simulink model "DroneSubsystem"  (R2018b)
settings: Solver=VariableStepAuto  StartTime=0.0  StopTime=10  RelTol=1e-3
values from neighbouring files (symbols this model uses):
  Ax = [0 1  0   0 ... (first row only)    [DroneSubsystemModelling.m]
  Ay = [0 1  0   0 ... (first row only)    [DroneSubsystemModelling.m]
  Bx = [0;0;0;b1]    [DroneSubsystemModelling.m]
  By = [0;0;0;b2]    [DroneSubsystemModelling.m]
  Cpx = [1 0 0 0]    [DroneSubsystemModelling.m]
  Cpy = [1 0 0 0]    [DroneSubsystemModelling.m]
  Cvx = [0 1 0 0]    [DroneSubsystemModelling.m]
  Cvy = [0 1 0 0]    [DroneSubsystemModelling.m]
  Dx = zeros(1,1)    [DroneSubsystemModelling.m]
  Dy = zeros(1,1)    [DroneSubsystemModelling.m]
  Ts = 0.001    [DroneSubsystemModelling.m]
  X40 = [x40 vx40 0 0]'    [MotionModelling.m]
  Y40 = [y40 vy40 0 0]'    [MotionModelling.m]
undefined symbols (not defined in the file or in its folder): x0, y0
libraries: simulink x6
settings Model: Creator=CowUser  LastModifiedBy=CowUser

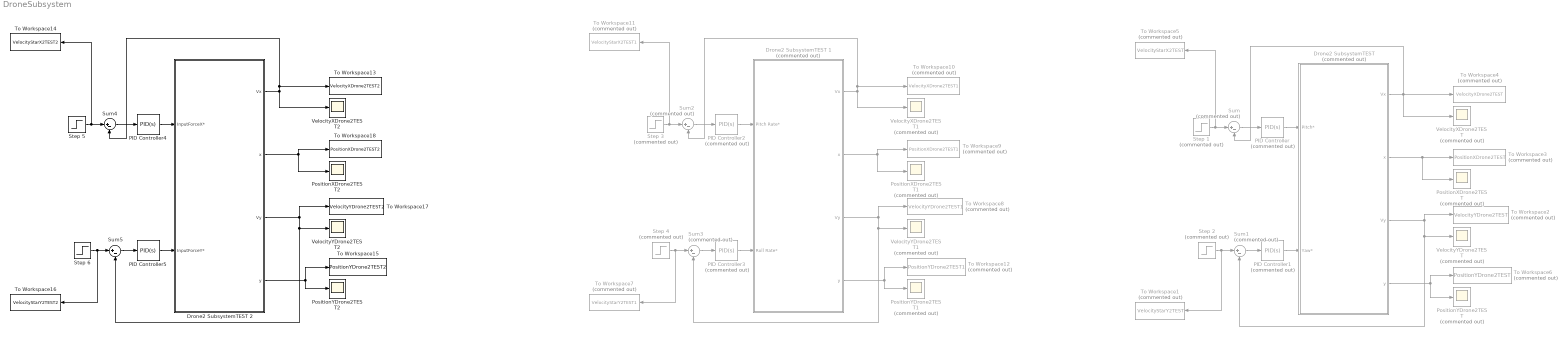
== system DroneSubsystem ==
  "Drone2 SubsystemTEST " : Subsystem  Commented=on
  Drone2 SubsystemTEST 1 : Subsystem  Commented=on
  Drone2 SubsystemTEST 2 : Subsystem
  PID Controller{,1..3} (4 alike) : simulink/Continuous/PID Controller  Commented=on  Controller=PID  Form=Parallel  TimeDomain=Continuous-time  SampleTime=-1  IntegratorMethod=Forward Euler  FilterMethod=Forward Euler  ControllerParametersSource=internal  P=800  I=40  D=1  UseFilter=on  N=100  TunerSelectOption=Transfer Function Based (PID Tuner App)  InitialConditionSource=internal  InitialConditionForIntegrator=0  InitialConditionForFilter=0  DifferentiatorICPrevScaledInput=0  ExternalReset=none  TrackingMode=off  Kt=1  LimitOutput=off  UpperSaturationLimit=inf  LowerSaturationLimit=-inf  LinearizeAsGain=on  AntiWindupMode=none  Kb=1  POutMin=[]  POutMax=[]  IOutMin=[]  IOutMax=[]  DOutMin=[]  DOutMax=[]  NOutMin=[]  NOutMax=[]  SumOutMin=[]  SumOutMax=[]  SaturationOutMin=[]  SaturationOutMax=[]  PParamMin=[]  PParamMax=[]  IParamMin=[]  IParamMax=[]  DParamMin=[]  DParamMax=[]  NParamMin=[]  NParamMax=[]  KbParamMin=[]  KbParamMax=[]  KtParamMin=[]  KtParamMax=[]  KbOutMin=[]  KbOutMax=[]  KtOutMin=[]  KtOutMax=[]  IntegratorOutMin=[]  IntegratorOutMax=[]  FilterOutMin=[]  FilterOutMax=[]  SumI1OutMin=[]  SumI1OutMax=[]  SumI2OutMin=[]  SumI2OutMax=[]  SumI3OutMin=[]  SumI3OutMax=[]  SumI4OutMin=[]  SumI4OutMax=[]  SumDOutMin=[]  SumDOutMax=[]  DifferentiatorOutMin=[]  DifferentiatorOutMax=[]  FilterDiffOutCoefMin=[]  FilterDiffOutCoefMax=[]  ReciprocalOutMin=[]  ReciprocalOutMax=[]  SumDenOutMin=[]  SumDenOutMax=[]  SumNumOutMin=[]  SumNumOutMax=[]  DivideOutMin=[]  DivideOutMax=[]  IntegratorContinuousStateAttributes=''  IntegratorStateMustResolveToSignalObject=off  IntegratorRTWStateStorageClass=Auto  FilterContinuousStateAttributes=''  FilterStateMustResolveToSignalObject=off  FilterRTWStateStorageClass=Auto  ParallelPVariant=InternalParameters  IdealPVariant=Disabled  IVariant=InternalParameters  DVariant=InternalParameters  IntegratorVariant=Continuous  SatVariant=Disabled  AWVariant=Passthrough  PCopyVariant=Disabled  TRVariant=Disabled  FdbkBlocksVariant=Forward  IdealPFdbkVariant=Disabled  SatFdbkVariant=Disabled  DerivativeFilterVariant=ContFilter  NVariant=InternalParameters  NCopyVariant=Disabled  FilterICVariant=InternalICsFilter  IntegratorICVariant=InternalICs  ExternalResetVariant=Disabled  TRSumVariant=Passthrough  SumFdbkVariant=Disabled  SumVariant=Sum_PID
  PID Controller4 : simulink/Continuous/PID Controller  Controller=PID  Form=Parallel  TimeDomain=Continuous-time  SampleTime=-1  IntegratorMethod=Forward Euler  FilterMethod=Forward Euler  ControllerParametersSource=internal  P=0.193233207738566  I=0.0113997087231983  D=0.323760304852997  UseFilter=on  N=866.923674741149  TunerSelectOption=Transfer Function Based (PID Tuner App)  InitialConditionSource=internal  InitialConditionForIntegrator=0  InitialConditionForFilter=0  DifferentiatorICPrevScaledInput=0  ExternalReset=none  TrackingMode=off  Kt=1  LimitOutput=off  UpperSaturationLimit=inf  LowerSaturationLimit=-inf  LinearizeAsGain=on  AntiWindupMode=none  Kb=1  POutMin=[]  POutMax=[]  IOutMin=[]  IOutMax=[]  DOutMin=[]  DOutMax=[]  NOutMin=[]  NOutMax=[]  SumOutMin=[]  SumOutMax=[]  SaturationOutMin=[]  SaturationOutMax=[]  PParamMin=[]  PParamMax=[]  IParamMin=[]  IParamMax=[]  DParamMin=[]  DParamMax=[]  NParamMin=[]  NParamMax=[]  KbParamMin=[]  KbParamMax=[]  KtParamMin=[]  KtParamMax=[]  KbOutMin=[]  KbOutMax=[]  KtOutMin=[]  KtOutMax=[]  IntegratorOutMin=[]  IntegratorOutMax=[]  FilterOutMin=[]  FilterOutMax=[]  SumI1OutMin=[]  SumI1OutMax=[]  SumI2OutMin=[]  SumI2OutMax=[]  SumI3OutMin=[]  SumI3OutMax=[]  SumI4OutMin=[]  SumI4OutMax=[]  SumDOutMin=[]  SumDOutMax=[]  DifferentiatorOutMin=[]  DifferentiatorOutMax=[]  FilterDiffOutCoefMin=[]  FilterDiffOutCoefMax=[]  ReciprocalOutMin=[]  ReciprocalOutMax=[]  SumDenOutMin=[]  SumDenOutMax=[]  SumNumOutMin=[]  SumNumOutMax=[]  DivideOutMin=[]  DivideOutMax=[]  IntegratorContinuousStateAttributes=''  IntegratorStateMustResolveToSignalObject=off  IntegratorRTWStateStorageClass=Auto  FilterContinuousStateAttributes=''  FilterStateMustResolveToSignalObject=off  FilterRTWStateStorageClass=Auto  ParallelPVariant=InternalParameters  IdealPVariant=Disabled  IVariant=InternalParameters  DVariant=InternalParameters  IntegratorVariant=Continuous  SatVariant=Disabled  AWVariant=Passthrough  PCopyVariant=Disabled  TRVariant=Disabled  FdbkBlocksVariant=Forward  IdealPFdbkVariant=Disabled  SatFdbkVariant=Disabled  DerivativeFilterVariant=ContFilter  NVariant=InternalParameters  NCopyVariant=Disabled  FilterICVariant=InternalICsFilter  IntegratorICVariant=InternalICs  ExternalResetVariant=Disabled  TRSumVariant=Passthrough  SumFdbkVariant=Disabled  SumVariant=Sum_PID
  PID Controller5 : simulink/Continuous/PID Controller  Controller=PID  Form=Parallel  TimeDomain=Continuous-time  SampleTime=-1  IntegratorMethod=Forward Euler  FilterMethod=Forward Euler  ControllerParametersSource=internal  P=1.97139727738968e-05  I=1.5233344900537e-08  D=0.00566857635684116  UseFilter=on  N=15.1370363747334  TunerSelectOption=Transfer Function Based (PID Tuner App)  InitialConditionSource=internal  InitialConditionForIntegrator=0  InitialConditionForFilter=0  DifferentiatorICPrevScaledInput=0  ExternalReset=none  TrackingMode=off  Kt=1  LimitOutput=off  UpperSaturationLimit=inf  LowerSaturationLimit=-inf  LinearizeAsGain=on  AntiWindupMode=none  Kb=1  POutMin=[]  POutMax=[]  IOutMin=[]  IOutMax=[]  DOutMin=[]  DOutMax=[]  NOutMin=[]  NOutMax=[]  SumOutMin=[]  SumOutMax=[]  SaturationOutMin=[]  SaturationOutMax=[]  PParamMin=[]  PParamMax=[]  IParamMin=[]  IParamMax=[]  DParamMin=[]  DParamMax=[]  NParamMin=[]  NParamMax=[]  KbParamMin=[]  KbParamMax=[]  KtParamMin=[]  KtParamMax=[]  KbOutMin=[]  KbOutMax=[]  KtOutMin=[]  KtOutMax=[]  IntegratorOutMin=[]  IntegratorOutMax=[]  FilterOutMin=[]  FilterOutMax=[]  SumI1OutMin=[]  SumI1OutMax=[]  SumI2OutMin=[]  SumI2OutMax=[]  SumI3OutMin=[]  SumI3OutMax=[]  SumI4OutMin=[]  SumI4OutMax=[]  SumDOutMin=[]  SumDOutMax=[]  DifferentiatorOutMin=[]  DifferentiatorOutMax=[]  FilterDiffOutCoefMin=[]  FilterDiffOutCoefMax=[]  ReciprocalOutMin=[]  ReciprocalOutMax=[]  SumDenOutMin=[]  SumDenOutMax=[]  SumNumOutMin=[]  SumNumOutMax=[]  DivideOutMin=[]  DivideOutMax=[]  IntegratorContinuousStateAttributes=''  IntegratorStateMustResolveToSignalObject=off  IntegratorRTWStateStorageClass=Auto  FilterContinuousStateAttributes=''  FilterStateMustResolveToSignalObject=off  FilterRTWStateStorageClass=Auto  ParallelPVariant=InternalParameters  IdealPVariant=Disabled  IVariant=InternalParameters  DVariant=InternalParameters  IntegratorVariant=Continuous  SatVariant=Disabled  AWVariant=Passthrough  PCopyVariant=Disabled  TRVariant=Disabled  FdbkBlocksVariant=Forward  IdealPFdbkVariant=Disabled  SatFdbkVariant=Disabled  DerivativeFilterVariant=ContFilter  NVariant=InternalParameters  NCopyVariant=Disabled  FilterICVariant=InternalICsFilter  IntegratorICVariant=InternalICs  ExternalResetVariant=Disabled  TRSumVariant=Passthrough  SumFdbkVariant=Disabled  SumVariant=Sum_PID
  PositionXDrone2TEST : Scope  Commented=on
  PositionXDrone2TEST1 : Scope  Commented=on
  PositionXDrone2TEST2 : Scope
  PositionYDrone2TEST : Scope  Commented=on
  PositionYDrone2TEST1 : Scope  Commented=on
  PositionYDrone2TEST2 : Scope
  Step {1..4} (4 alike) : Step  Commented=on  Time=0  After=-0.1061  SampleTime=0
  Step 5 : Step  Time=0  After=0.1061  SampleTime=0
  Step 6 : Step  Time=0  After=0.1061  SampleTime=0
  Sum{,1..3} (4 alike) : Sum  Commented=on  Inputs=|+-
  Sum4 : Sum  Inputs=|+-
  Sum5 : Sum  Inputs=|+-
  To Workspace1 : ToWorkspace  Commented=on  VariableName=VelocityStarY2TEST  SampleTime=-1
  To Workspace10 : ToWorkspace  Commented=on  VariableName=VelocityXDrone2TEST1  SampleTime=-1
  To Workspace11 : ToWorkspace  Commented=on  VariableName=VelocityStarX2TEST1  SampleTime=-1
  To Workspace12 : ToWorkspace  Commented=on  VariableName=PositionYDrone2TEST1  SampleTime=-1
  To Workspace13 : ToWorkspace  VariableName=VelocityXDrone2TEST2  SampleTime=-1
  To Workspace14 : ToWorkspace  VariableName=VelocityStarX2TEST2  SampleTime=-1
  To Workspace15 : ToWorkspace  VariableName=PositionYDrone2TEST2  SampleTime=-1
  To Workspace16 : ToWorkspace  VariableName=VelocityStarY2TEST2  SampleTime=-1
  To Workspace17 : ToWorkspace  VariableName=VelocityYDrone2TEST2  SampleTime=-1
  To Workspace18 : ToWorkspace  VariableName=PositionXDrone2TEST2  SampleTime=-1
  To Workspace2 : ToWorkspace  Commented=on  VariableName=VelocityYDrone2TEST  SampleTime=-1
  To Workspace3 : ToWorkspace  Commented=on  VariableName=PositionXDrone2TEST  SampleTime=-1
  To Workspace4 : ToWorkspace  Commented=on  VariableName=VelocityXDrone2TEST  SampleTime=-1
  To Workspace5 : ToWorkspace  Commented=on  VariableName=VelocityStarX2TEST  SampleTime=-1
  To Workspace6 : ToWorkspace  Commented=on  VariableName=PositionYDrone2TEST  SampleTime=-1
  To Workspace7 : ToWorkspace  Commented=on  VariableName=VelocityStarY2TEST1  SampleTime=-1
  To Workspace8 : ToWorkspace  Commented=on  VariableName=VelocityYDrone2TEST1  SampleTime=-1
  To Workspace9 : ToWorkspace  Commented=on  VariableName=PositionXDrone2TEST1  SampleTime=-1
  VelocityXDrone2TEST : Scope  Commented=on
  VelocityXDrone2TEST1 : Scope  Commented=on
  VelocityXDrone2TEST2 : Scope
  VelocityYDrone2TEST : Scope  Commented=on
  VelocityYDrone2TEST1 : Scope  Commented=on
  VelocityYDrone2TEST2 : Scope
  wires:
  Step 2/1 -> To Workspace1/1, Sum1/1
  "Drone2 SubsystemTEST "/2(x) -> To Workspace3/1, PositionXDrone2TEST/1
  Sum1/1 -> PID Controller1/1
  PID Controller/1 -> "Drone2 SubsystemTEST "/1(Pitch*)
  Sum/1 -> PID Controller/1
  "Drone2 SubsystemTEST "/4(y) -> To Workspace6/1, PositionYDrone2TEST/1
  PID Controller1/1 -> "Drone2 SubsystemTEST "/2("Yaw* ")
  Step 1/1 -> Sum/1, To Workspace5/1
  "Drone2 SubsystemTEST "/3(Vy) -> To Workspace2/1, Sum1/2, VelocityYDrone2TEST/1
  "Drone2 SubsystemTEST "/1(Vx) -> VelocityXDrone2TEST/1, Sum/2, To Workspace4/1
  Sum3/1 -> PID Controller3/1
  Step 4/1 -> To Workspace7/1, Sum3/1
  Step 3/1 -> Sum2/1, To Workspace11/1
  PID Controller3/1 -> Drone2 SubsystemTEST 1/2("Roll Rate* ")
  Drone2 SubsystemTEST 1/1(Vx) -> Sum2/2, To Workspace10/1, VelocityXDrone2TEST1/1
  Drone2 SubsystemTEST 1/4(y) -> To Workspace12/1, PositionYDrone2TEST1/1
  Drone2 SubsystemTEST 1/2(x) -> To Workspace9/1, PositionXDrone2TEST1/1
  Drone2 SubsystemTEST 1/3(Vy) -> Sum3/2, VelocityYDrone2TEST1/1, To Workspace8/1
  Sum2/1 -> PID Controller2/1
  PID Controller2/1 -> Drone2 SubsystemTEST 1/1(Pitch Rate*)
  Sum4/1 -> PID Controller4/1
  Drone2 SubsystemTEST 2/1(Vx) -> Sum4/2, To Workspace13/1, VelocityXDrone2TEST2/1
  Drone2 SubsystemTEST 2/2(x) -> To Workspace18/1, PositionXDrone2TEST2/1
  PID Controller4/1 -> Drone2 SubsystemTEST 2/1(InputForceX*)
  Step 5/1 -> Sum4/1, To Workspace14/1
  Sum5/1 -> PID Controller5/1
  Drone2 SubsystemTEST 2/3(Vy) -> Sum5/2, VelocityYDrone2TEST2/1, To Workspace17/1
  Drone2 SubsystemTEST 2/4(y) -> To Workspace15/1, PositionYDrone2TEST2/1
  Step 6/1 -> To Workspace16/1, Sum5/1
  PID Controller5/1 -> Drone2 SubsystemTEST 2/2("InputForceY* ")

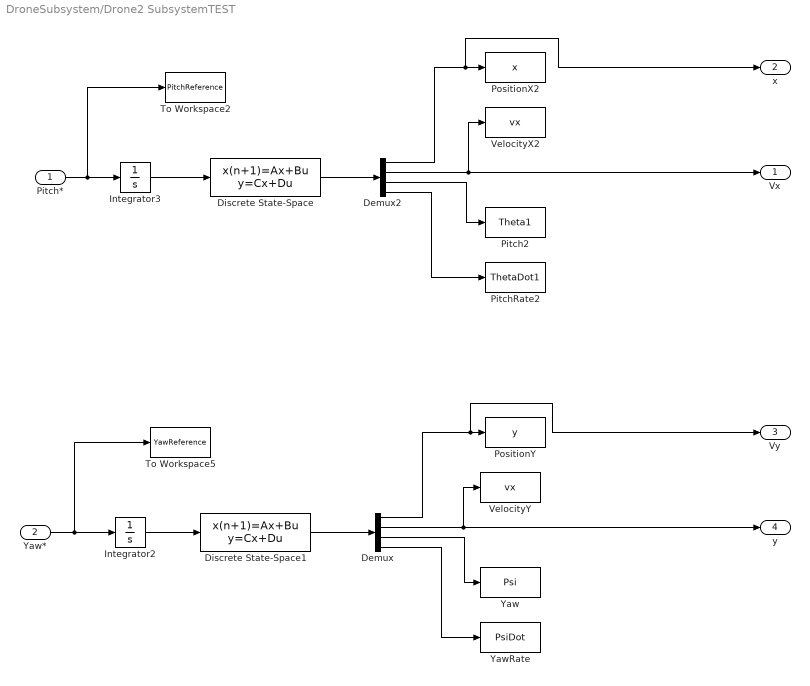
== system DroneSubsystem/Drone2 SubsystemTEST  ==
  Pitch* : Inport
  "Yaw* " : Inport  Port=2
  Demux : Demux
  Demux2 : Demux
  Discrete State-Space : DiscreteStateSpace  A=Ax  B=Bx  C=Cvx  D=Dx  InitialCondition=x0  SampleTime=Ts
  Discrete State-Space1 : DiscreteStateSpace  A=Ay  B=By  C=Cvy  D=Dy  InitialCondition=y0  SampleTime=Ts
  Integrator2 : Integrator
  Integrator3 : Integrator
  Pitch2 : ToWorkspace  VariableName=Theta1  SampleTime=-1
  PitchRate2 : ToWorkspace  VariableName=ThetaDot1  SampleTime=-1
  PositionX2 : ToWorkspace  VariableName=x  SampleTime=-1
  PositionY : ToWorkspace  VariableName=y  SampleTime=-1
  To Workspace2 : ToWorkspace  VariableName=PitchReference  SampleTime=-1
  To Workspace5 : ToWorkspace  VariableName=YawReference  SampleTime=-1
  VelocityX2 : ToWorkspace  VariableName=vx  SampleTime=-1
  VelocityY : ToWorkspace  VariableName=vx  SampleTime=-1
  Yaw : ToWorkspace  VariableName=Psi  SampleTime=-1
  YawRate : ToWorkspace  VariableName=PsiDot  SampleTime=-1
  Vx : Outport
  x : Outport  Port=2
  Vy : Outport  Port=3
  y : Outport  Port=4
  wires:
  Integrator3/1 -> Discrete State-Space/1
  Pitch*/1 -> Integrator3/1, To Workspace2/1
  Demux2/3 -> Pitch2/1
  Discrete State-Space/1 -> Demux2/1
  Demux2/4 -> PitchRate2/1
  Integrator2/1 -> Discrete State-Space1/1
  "Yaw* "/1 -> Integrator2/1, To Workspace5/1
  Demux/3 -> Yaw/1
  Discrete State-Space1/1 -> Demux/1
  Demux/4 -> YawRate/1
  Demux2/2 -> Vx/1, VelocityX2/1
  Demux2/1 -> x/1, PositionX2/1
  Demux/2 -> VelocityY/1, y/1
  Demux/1 -> Vy/1, PositionY/1

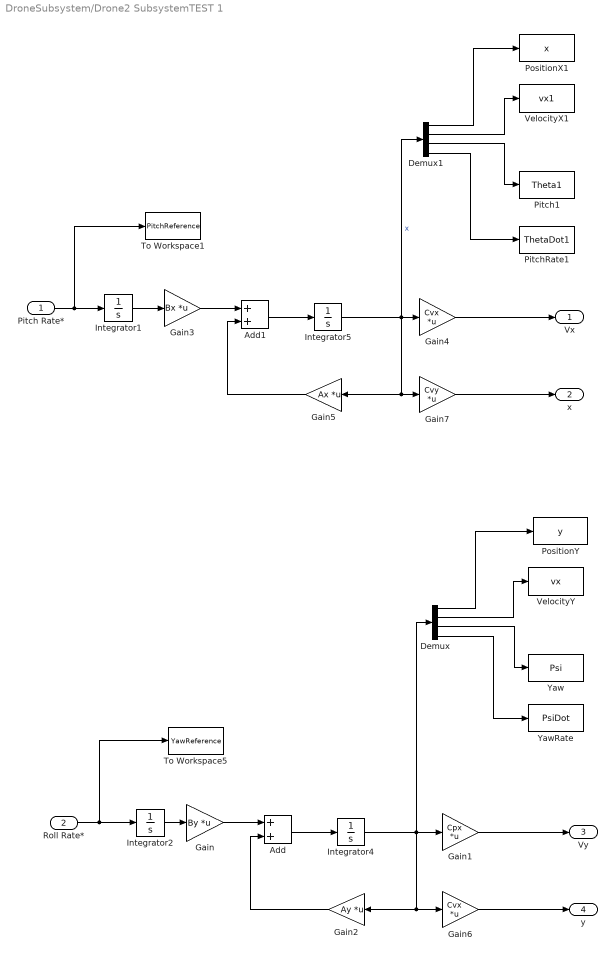
== system DroneSubsystem/Drone2 SubsystemTEST 1 ==
  Pitch Rate* : Inport
  "Roll Rate* " : Inport  Port=2
  Add : Sum
  Add1 : Sum
  Demux : Demux
  Demux1 : Demux
  Gain : Gain  Gain=By  Multiplication=Matrix(K*u)
  Gain1 : Gain  Gain=Cpx  Multiplication=Matrix(K*u)
  Gain2 : Gain  Gain=Ay  Multiplication=Matrix(K*u)
  Gain3 : Gain  Gain=Bx  Multiplication=Matrix(K*u)
  Gain4 : Gain  Gain=Cvx  Multiplication=Matrix(K*u)
  Gain5 : Gain  Gain=Ax  Multiplication=Matrix(K*u)
  Gain6 : Gain  Gain=Cvx  Multiplication=Matrix(K*u)
  Gain7 : Gain  Gain=Cvy  Multiplication=Matrix(K*u)
  Integrator1 : Integrator
  Integrator2 : Integrator
  Integrator4 : Integrator  InitialCondition=y0
  Integrator5 : Integrator  InitialCondition=x0
  Pitch1 : ToWorkspace  VariableName=Theta1  SampleTime=-1
  PitchRate1 : ToWorkspace  VariableName=ThetaDot1  SampleTime=-1
  PositionX1 : ToWorkspace  VariableName=x  SampleTime=-1
  PositionY : ToWorkspace  VariableName=y  SampleTime=-1
  To Workspace1 : ToWorkspace  VariableName=PitchReference  SampleTime=-1
  To Workspace5 : ToWorkspace  VariableName=YawReference  SampleTime=-1
  VelocityX1 : ToWorkspace  VariableName=vx1  SampleTime=-1
  VelocityY : ToWorkspace  VariableName=vx  SampleTime=-1
  Yaw : ToWorkspace  VariableName=Psi  SampleTime=-1
  YawRate : ToWorkspace  VariableName=PsiDot  SampleTime=-1
  Vx : Outport
  x : Outport  Port=2
  Vy : Outport  Port=3
  y : Outport  Port=4
  wires:
  Demux1/4 -> PitchRate1/1
  Demux1/2 -> VelocityX1/1
  Integrator2/1 -> Gain/1
  Gain4/1 -> Vx/1
  Integrator1/1 -> Gain3/1
  Integrator4/1 -> Gain6/1, Gain2/1, Demux/1, Gain1/1
  Integrator5/1 -> Gain4/1, Gain5/1, Gain7/1, Demux1/1  "x"
  Add1/1 -> Integrator5/1
  Gain5/1 -> Add1/2
  Demux1/3 -> Pitch1/1
  Gain3/1 -> Add1/1
  Gain7/1 -> x/1
  Pitch Rate*/1 -> Integrator1/1, To Workspace1/1
  Gain2/1 -> Add/2
  Demux/2 -> VelocityY/1
  Gain1/1 -> Vy/1
  Add/1 -> Integrator4/1
  Demux1/1 -> PositionX1/1
  Gain6/1 -> y/1
  Demux/3 -> Yaw/1
  Demux/1 -> PositionY/1
  "Roll Rate* "/1 -> Integrator2/1, To Workspace5/1
  Gain/1 -> Add/1
  Demux/4 -> YawRate/1

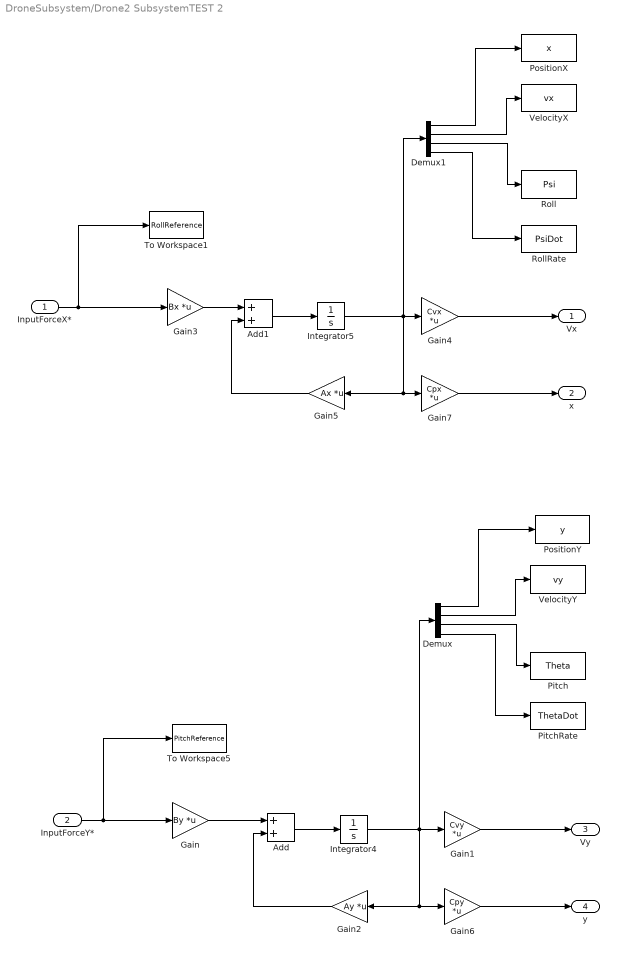
== system DroneSubsystem/Drone2 SubsystemTEST 2 ==
  InputForceX* : Inport
  "InputForceY* " : Inport  Port=2
  Add : Sum
  Add1 : Sum
  Demux : Demux
  Demux1 : Demux
  Gain : Gain  Gain=By  Multiplication=Matrix(K*u)
  Gain1 : Gain  Gain=Cvy  Multiplication=Matrix(K*u)
  Gain2 : Gain  Gain=Ay  Multiplication=Matrix(K*u)
  Gain3 : Gain  Gain=Bx  Multiplication=Matrix(K*u)
  Gain4 : Gain  Gain=Cvx  Multiplication=Matrix(K*u)
  Gain5 : Gain  Gain=Ax  Multiplication=Matrix(K*u)
  Gain6 : Gain  Gain=Cpy  Multiplication=Matrix(K*u)
  Gain7 : Gain  Gain=Cpx  Multiplication=Matrix(K*u)
  Integrator4 : Integrator  InitialCondition=Y40
  Integrator5 : Integrator  InitialCondition=X40
  Pitch : ToWorkspace  VariableName=Theta  SampleTime=-1
  PitchRate : ToWorkspace  VariableName=ThetaDot  SampleTime=-1
  PositionX : ToWorkspace  VariableName=x  SampleTime=-1
  PositionY : ToWorkspace  VariableName=y  SampleTime=-1
  Roll : ToWorkspace  VariableName=Psi  SampleTime=-1
  RollRate : ToWorkspace  VariableName=PsiDot  SampleTime=-1
  To Workspace1 : ToWorkspace  VariableName=RollReference  SampleTime=-1
  To Workspace5 : ToWorkspace  VariableName=PitchReference  SampleTime=-1
  VelocityX : ToWorkspace  VariableName=vx  SampleTime=-1
  VelocityY : ToWorkspace  VariableName=vy  SampleTime=-1
  Vx : Outport
  x : Outport  Port=2
  Vy : Outport  Port=3
  y : Outport  Port=4
  wires:
  Demux1/4 -> RollRate/1
  Demux1/2 -> VelocityX/1
  Gain4/1 -> Vx/1
  Integrator4/1 -> Gain6/1, Gain2/1, Demux/1, Gain1/1
  Integrator5/1 -> Gain4/1, Gain5/1, Gain7/1, Demux1/1
  Add1/1 -> Integrator5/1
  Gain5/1 -> Add1/2
  Demux1/3 -> Roll/1
  Gain3/1 -> Add1/1
  Gain7/1 -> x/1
  Gain2/1 -> Add/2
  Demux/2 -> VelocityY/1
  Gain1/1 -> Vy/1
  Add/1 -> Integrator4/1
  Demux1/1 -> PositionX/1
  Gain6/1 -> y/1
  Demux/3 -> Pitch/1
  Demux/1 -> PositionY/1
  Gain/1 -> Add/1
  Demux/4 -> PitchRate/1
  "InputForceY* "/1 -> Gain/1, To Workspace5/1
  InputForceX*/1 -> Gain3/1, To Workspace1/1
